simulink subsystem "Day2_Scenario_4_5"  (R2024a)
settings: Solver=VariableStepAuto  StartTime=0.0  StopTime=10.0  RelTol=1e-3
undefined symbols (not defined in the file): route1_waypoint_raw
libraries: CarMaker4SL x6, slpidlib x1
settings Model: Creator=junhyung.cha  LastModifiedBy=hajin

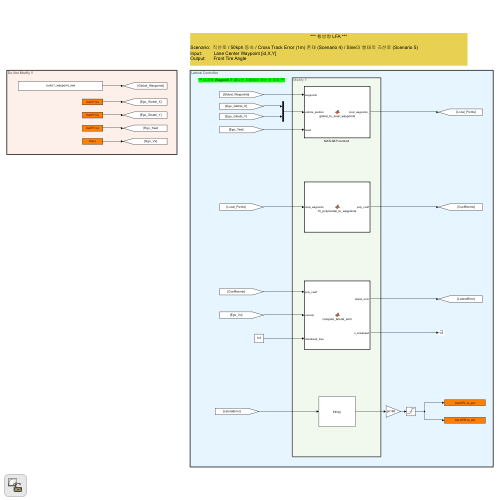
[thumbnail: Simulink's stored preview of the top-level diagram]
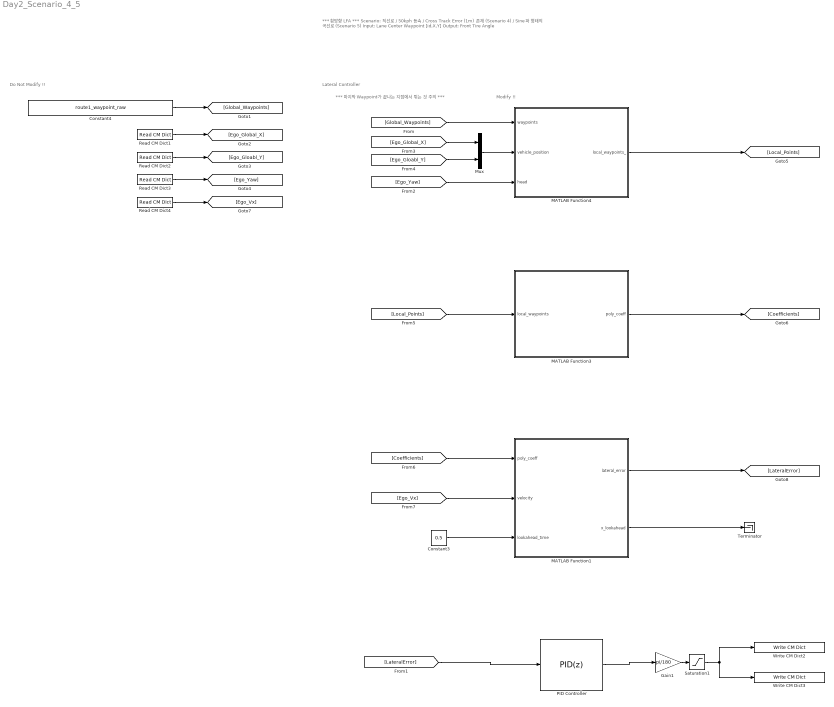
== system Day2_Scenario_4_5 ==
  note: *** 마지막 Waypoint가 끝나는 지점에서 튀는 것 주의 ***
  note: Modify !!
  note: Lateral Controller
  note: Do Not Modify !!
  note: *** 횡방향 LFA ***
      |
      | Scenario: 직선로 / 50kph 등속 / Cross Track Error (1m) 존재 (Scenario 4) / Sine파 형태의 곡선로 (Scenario 5)
      | Input: Lane Center Waypoint [id,X,Y]
      | Output: Front Tire Angle
  Constant3 : Constant  Value=0.5
  Constant4 : Constant  Value=route1_waypoint_raw
  Gain1 : Gain  Gain=pi/180
  MATLAB Function1 : MATLAB Function  TreatAsAtomicUnit=on
  MATLAB Function3 : MATLAB Function  TreatAsAtomicUnit=on
  "MATLAB Function4 " : MATLAB Function  TreatAsAtomicUnit=on
  Mux : Mux  Inputs=2
  PID Controller : slpidlib/PID Controller  Controller=PID  Form=Parallel  TimeDomain=Discrete-time  UseExternalTs=off  SampleTime=-1  IntegratorMethod=Forward Euler  FilterMethod=Forward Euler  ControllerParametersSource=internal  P=8  I=0  UseKiTs=off  D=0.5  UseExternalDerivativeSource=off  N=100  UseFilter=on  TunerSelectOption=Transfer Function Based (PID Tuner App)  InitialConditionSource=internal  InitialConditionForIntegrator=0  InitialConditionForFilter=0  DifferentiatorICPrevScaledInput=0  ExternalReset=none  TrackingMode=off  Kt=1  LimitOutput=off  SatLimitsSource=internal  UpperSaturationLimit=inf  LowerSaturationLimit=-inf  LinearizeAsGain=on  AntiWindupMode=none  Kb=1  LimitIntegrator=off  UpperIntegratorSaturationLimit=inf  LowerIntegratorSaturationLimit=-inf  POutMin=[]  POutMax=[]  IOutMin=[]  IOutMax=[]  DOutMin=[]  DOutMax=[]  NOutMin=[]  NOutMax=[]  SumOutMin=[]  SumOutMax=[]  SaturationOutMin=[]  SaturationOutMax=[]  PParamMin=[]  PParamMax=[]  IParamMin=[]  IParamMax=[]  DParamMin=[]  DParamMax=[]  NParamMin=[]  NParamMax=[]  KbParamMin=[]  KbParamMax=[]  KtParamMin=[]  KtParamMax=[]  KbOutMin=[]  KbOutMax=[]  KtOutMin=[]  KtOutMax=[]  IntegratorOutMin=[]  IntegratorOutMax=[]  FilterOutMin=[]  FilterOutMax=[]  SumI1OutMin=[]  SumI1OutMax=[]  SumI2OutMin=[]  SumI2OutMax=[]  SumI3OutMin=[]  SumI3OutMax=[]  SumI4OutMin=[]  SumI4OutMax=[]  SumDOutMin=[]  SumDOutMax=[]  DifferentiatorOutMin=[]  DifferentiatorOutMax=[]  FilterDiffOutCoefMin=[]  FilterDiffOutCoefMax=[]  ReciprocalOutMin=[]  ReciprocalOutMax=[]  SumDenOutMin=[]  SumDenOutMax=[]  SumNumOutMin=[]  SumNumOutMax=[]  DivideOutMin=[]  DivideOutMax=[]  UdiffTsProdOutMin=[]  UdiffTsProdOutMax=[]  NTsProdOutMin=[]  NTsProdOutMax=[]  UintegralTsProdOutMin=[]  UintegralTsProdOutMax=[]  UngainTsProdOutMin=[]  UngainTsProdOutMax=[]  ClampingZeroOutDataTypeStr=Inherit: Inherit via back propagation  ClampingZeroOutMin=[]  ClampingZeroOutMax=[]  FilterDenConstantOutDataTypeStr=Inherit: Inherit via back propagation  FilterDenConstantOutMin=[]  FilterDenConstantOutMax=[]  PCopyOutDataTypeStr=Inherit: Inherit via back propagation  PCopyOutMin=[]  PCopyOutMax=[]  NCopyOutDataTypeStr=Inherit: Inherit via back propagation  NCopyOutMin=[]  NCopyOutMax=[]  IntegratorContinuousStateAttributes=''  IntegratorStateMustResolveToSignalObject=off  IntegratorRTWStateStorageClass=Auto  FilterContinuousStateAttributes=''  FilterStateMustResolveToSignalObject=off  FilterRTWStateStorageClass=Auto  ParallelPVariant=InternalParameters  IdealPVariant=Disabled  IVariant=InternalParameters  DVariant=InternalParameters  IntegratorVariant=Discrete  SatVariant=Disabled  AWVariant=Passthrough  PCopyVariant=Disabled  TRVariant=Disabled  FdbkBlocksVariant=Forward  IdealPFdbkVariant=Disabled  SatFdbkVariant=Disabled  DerivativeFilterVariant=ForwardEulerFilter  NVariant=InternalParameters  NCopyVariant=Disabled  FilterICVariant=InternalICsFilter  IntegratorICVariant=InternalICs  ExternalResetVariant=Disabled  TRSumVariant=Passthrough  SumFdbkVariant=Disabled  SumVariant=Sum_PID  TsampFilterVariant=InternalTs  TsampNgainVariant=Passthrough  TsampIntegralVariant=Disabled_SignalSpec  ExternalSaturationOutDataTypeStr=Inherit: Same as second input  DerivativeSourceVariant=ErrorSignal
  Read CM Dict1 : CarMaker4SL/Read CM Dict  xname=Car.Fr1.tx  xsync=off  xstime=Inherited
  Read CM Dict2 : CarMaker4SL/Read CM Dict  xname=Car.Fr1.ty  xsync=off  xstime=Inherited
  Read CM Dict3 : CarMaker4SL/Read CM Dict  xname=Car.Fr1.rz  xsync=off  xstime=Inherited
  Read CM Dict4 : CarMaker4SL/Read CM Dict  xname=Car.v  xsync=off  xstime=Inherited
  Saturation1 : Saturate  UpperLimit=2  LowerLimit=-2
  Terminator : Terminator
  Write CM Dict2 : CarMaker4SL/Write CM Dict  xname=Car.CFL.rz_ext  xsync=off
  Write CM Dict3 : CarMaker4SL/Write CM Dict  xname=Car.CFR.rz_ext  xsync=off
  wires:
  Read CM Dict1/1 -> [Ego_Global_X]
  Read CM Dict2/1 -> [Ego_Gloabl_Y]
  Read CM Dict3/1 -> [Ego_Yaw]
  [Ego_Yaw] -> "MATLAB Function4 "/3(head)
  [Ego_Global_X] -> Mux/1
  [Ego_Gloabl_Y] -> Mux/2
  "MATLAB Function4 "/1(local_waypoints_) -> [Local_Points]
  [Global_Waypoints] -> "MATLAB Function4 "/1(waypoints)
  [Local_Points] -> MATLAB Function3/1(local_waypoints)
  MATLAB Function3/1(poly_coeff) -> [Coefficients]
  [Coefficients] -> MATLAB Function1/1(poly_coeff)
  Constant3/1 -> MATLAB Function1/3(lookahead_time)
  Saturation1/1 -> Write CM Dict3/1, Write CM Dict2/1
  MATLAB Function1/1(lateral_error) -> [LateralError]
  [LateralError] -> PID Controller/1
  [Ego_Vx] -> MATLAB Function1/2(velocity)
  Constant4/1 -> [Global_Waypoints]
  PID Controller/1 -> Gain1/1
  Gain1/1 -> Saturation1/1
  Mux/1 -> "MATLAB Function4 "/2(vehicle_position)
  MATLAB Function1/2(x_lookahead) -> Terminator/1
  Read CM Dict4/1 -> [Ego_Vx]

== matlab function Day2_Scenario_4_5/MATLAB Function1 ==
  settings: updateMethod=DISCRETE  sampleTime=0.05
  data: poly_coeff input; lateral_error output; velocity input; lookahead_time input; x_lookahead output
function [lateral_error, x_lookahead] = compute_lateral_error(poly_coeff, velocity, lookahead_time)

persistent err_prev
if isempty(err_prev)
    err_prev = 0;
end

x_lookahead = velocity * lookahead_time;
raw_err = polyval(poly_coeff, x_lookahead);

% NaN/inf 안전장치
if ~isfinite(raw_err)
    raw_err = 0;
end
% 절대값 제한
if raw_err > 5, raw_err = 5; end
if raw_err < -5, raw_err = -5; end

% 저역통과 필터 (α=0.4: 노이즈 억제)
alpha = 0.4;
lateral_error = alpha * raw_err + (1 - alpha) * err_prev;
err_prev = lateral_error;

end

== matlab function Day2_Scenario_4_5/MATLAB Function3 ==
  settings: updateMethod=DISCRETE  sampleTime=0.05
  data: local_waypoints input; poly_coeff output
function poly_coeff = fit_polynomial_to_waypoints(local_waypoints)

% local_waypoints: Nx2 [X_local, Y_local]
% 적응형 차수: 곡선이면 3차, 직선이면 1차 자동 선택

N_pts = size(local_waypoints, 1);
x = local_waypoints(:, 1);
y = local_waypoints(:, 2);

% 가장 가까운 웨이포인트
dist_sq = x.^2 + y.^2;
[~, i_min] = min(dist_sq);

% 윈도우: 25점 (곡선 추종 + 노이즈 억제 균형)
N_window = 25;
i_end = min(i_min + N_window, N_pts);
seg_x = x(i_min:i_end);
seg_y = y(i_min:i_end);

sel = seg_x > 0;
x_fwd = seg_x(sel);
y_fwd = seg_y(sel);

poly_coeff = [0 0 0 0];
if numel(x_fwd) >= 5 && (max(x_fwd) - min(x_fwd)) > 2
    % 로컬 y 변동 측정: 곡선이면 크고, 직선이면 작음
    y_range = max(y_fwd) - min(y_fwd);
    if y_range > 0.5
        % 곡선: 3차 다항식
        poly_coeff = polyfit(x_fwd, y_fwd, 3);
    else
        % 거의 직선: 1차 피팅 (노이즈 억제)
        c = polyfit(x_fwd, y_fwd, 1);
        poly_coeff = [0, 0, c(1), c(2)];
    end
end

% NaN/inf 안전장치
for k = 1:4
    if ~isfinite(poly_coeff(k))
        poly_coeff = [0 0 0 0];
        break;
    end
end

end

== matlab function Day2_Scenario_4_5/MATLAB Function4  ==
  settings: updateMethod=DISCRETE  sampleTime=0.05
  data: waypoints input; local_waypoints_ output; vehicle_position input; head input
function local_waypoints_ = global_to_local_waypoints(waypoints, vehicle_position, head)

% waypoints: Nx2 행렬 [X_global, Y_global]
% vehicle_position: [X; Y] 글로벌 좌표
% head: 차량 yaw 각도 [rad]

N = size(waypoints, 1);
local_waypoints_ = zeros(N, 2);

cos_h = cos(head);
sin_h = sin(head);

for i = 1:N
    dx = waypoints(i, 1) - vehicle_position(1);
    dy = waypoints(i, 2) - vehicle_position(2);

    % -head 만큼 회전 (글로벌 -> 차량 로컬)
    local_waypoints_(i, 1) =  cos_h * dx + sin_h * dy;
    local_waypoints_(i, 2) = -sin_h * dx + cos_h * dy;
end

end
